simulink model "simulink_guidance_system"  (R2025a)
settings: Solver=VariableStepAuto  StartTime=0.0  StopTime=231  RelTol=1e-3
libraries: slpidlib x1
settings Model: Creator=javia  LastModifiedBy=javia

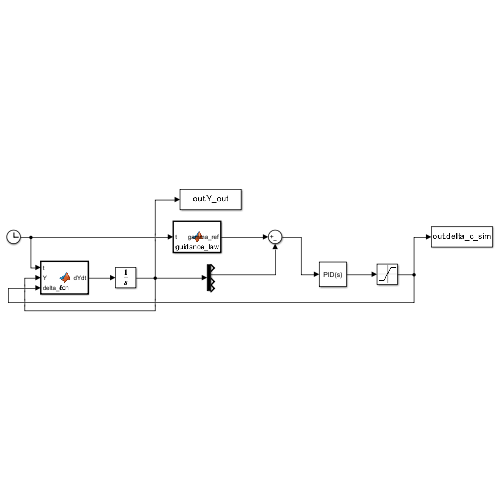
[thumbnail: Simulink's stored preview of the top-level diagram]
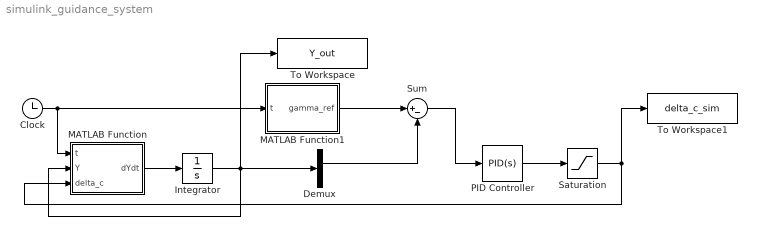
== system simulink_guidance_system ==
  Clock : Clock
  Demux : Demux
  Integrator : Integrator  InitialCondition=[0; pi/2; 0; 0]
  MATLAB Function : MATLAB Function  TreatAsAtomicUnit=on
  MATLAB Function1 : MATLAB Function  TreatAsAtomicUnit=on
  PID Controller : slpidlib/PID Controller  Controller=PID  Form=Parallel  TimeDomain=Continuous-time  UseExternalTs=off  SampleTime=-1  IntegratorMethod=Forward Euler  FilterMethod=Forward Euler  ControllerParametersSource=internal  P=3  I=0.5  UseKiTs=off  D=2  UseExternalDerivativeSource=off  N=100  UseFilter=on  TunerSelectOption=Transfer Function Based (PID Tuner App)  InitialConditionSource=internal  InitialConditionForIntegrator=0  InitialConditionForFilter=0  DifferentiatorICPrevScaledInput=0  ExternalReset=none  TrackingMode=off  Kt=1  LimitOutput=off  SatLimitsSource=internal  UpperSaturationLimit=10 * (pi/180)  LowerSaturationLimit=-10 * (pi/180)  LinearizeAsGain=on  AntiWindupMode=clamping  Kb=1  LimitIntegrator=off  UpperIntegratorSaturationLimit=inf  LowerIntegratorSaturationLimit=-inf  POutMin=[]  POutMax=[]  IOutMin=[]  IOutMax=[]  DOutMin=[]  DOutMax=[]  NOutMin=[]  NOutMax=[]  SumOutMin=[]  SumOutMax=[]  SaturationOutMin=[]  SaturationOutMax=[]  PParamMin=[]  PParamMax=[]  IParamMin=[]  IParamMax=[]  DParamMin=[]  DParamMax=[]  NParamMin=[]  NParamMax=[]  KbParamMin=[]  KbParamMax=[]  KtParamMin=[]  KtParamMax=[]  KbOutMin=[]  KbOutMax=[]  KtOutMin=[]  KtOutMax=[]  IntegratorOutMin=[]  IntegratorOutMax=[]  FilterOutMin=[]  FilterOutMax=[]  SumI1OutMin=[]  SumI1OutMax=[]  SumI2OutMin=[]  SumI2OutMax=[]  SumI3OutMin=[]  SumI3OutMax=[]  SumI4OutMin=[]  SumI4OutMax=[]  SumDOutMin=[]  SumDOutMax=[]  DifferentiatorOutMin=[]  DifferentiatorOutMax=[]  FilterDiffOutCoefMin=[]  FilterDiffOutCoefMax=[]  ReciprocalOutMin=[]  ReciprocalOutMax=[]  SumDenOutMin=[]  SumDenOutMax=[]  SumNumOutMin=[]  SumNumOutMax=[]  DivideOutMin=[]  DivideOutMax=[]  UdiffTsProdOutMin=[]  UdiffTsProdOutMax=[]  NTsProdOutMin=[]  NTsProdOutMax=[]  UintegralTsProdOutMin=[]  UintegralTsProdOutMax=[]  UngainTsProdOutMin=[]  UngainTsProdOutMax=[]  ClampingZeroOutDataTypeStr=Inherit: Inherit via back propagation  ClampingZeroOutMin=[]  ClampingZeroOutMax=[]  FilterDenConstantOutDataTypeStr=Inherit: Inherit via back propagation  FilterDenConstantOutMin=[]  FilterDenConstantOutMax=[]  PCopyOutDataTypeStr=Inherit: Inherit via back propagation  PCopyOutMin=[]  PCopyOutMax=[]  NCopyOutDataTypeStr=Inherit: Inherit via back propagation  NCopyOutMin=[]  NCopyOutMax=[]  IntegratorContinuousStateAttributes=''  IntegratorStateMustResolveToSignalObject=off  IntegratorRTWStateStorageClass=Auto  FilterContinuousStateAttributes=''  FilterStateMustResolveToSignalObject=off  FilterRTWStateStorageClass=Auto  ParallelPVariant=InternalParameters  IdealPVariant=Disabled  IVariant=InternalParameters  DVariant=InternalParameters  IntegratorVariant=Continuous  SatVariant=Disabled  AWVariant=Passthrough  PCopyVariant=Disabled  TRVariant=Disabled  FdbkBlocksVariant=Forward  IdealPFdbkVariant=Disabled  SatFdbkVariant=Disabled  DerivativeFilterVariant=ContFilter  NVariant=InternalParameters  NCopyVariant=Disabled  FilterICVariant=InternalICsFilter  IntegratorICVariant=InternalICs  ExternalResetVariant=Disabled  TRSumVariant=Passthrough  SumFdbkVariant=Disabled  SumVariant=Sum_PID  TsampFilterVariant=InternalTs  TsampNgainVariant=Passthrough  TsampIntegralVariant=Passthrough  ExternalSaturationOutDataTypeStr=Inherit: Same as second input  DerivativeSourceVariant=ErrorSignal  PreIntVariant=InternalPreInt
  Saturation : Saturate  UpperLimit=10 * (pi/180)  LowerLimit=-10 * (pi/180)
  Sum : Sum  Inputs=|+-
  To Workspace : ToWorkspace  VariableName=Y_out  SampleTime=-1
  To Workspace1 : ToWorkspace  VariableName=delta_c_sim  SampleTime=-1
  wires:
  Clock/1 -> MATLAB Function1/1(t), MATLAB Function/1(t)
  MATLAB Function/1(dYdt) -> Integrator/1
  Integrator/1 -> MATLAB Function/2(Y), To Workspace/1, Demux/1
  MATLAB Function1/1(gamma_ref) -> Sum/1
  Demux/2 -> Sum/2
  Sum/1 -> PID Controller/1
  PID Controller/1 -> Saturation/1
  Saturation/1 -> MATLAB Function/3(delta_c), To Workspace1/1

== matlab function simulink_guidance_system/MATLAB Function ==
  data: t input; dYdt output; Y input; delta_c input
function dYdt = fcn(t, Y, delta_c)
    % Obtain current State Vector values
    V = Y(1);
    gamma = Y(2);
    z = Y(3);
    psi = Y(4);
    
    Rt = 6378140;  % Earth mean radius [m]
    
    % Call parameters from your modular files
    [m_t0, tb_1, mass_flow1, T1] = f_stage1();
    [t_GT, ~] = f_gravity_turn();
    [T2, mass_flow2, m0_phase3, tb_2] = f_stage2();
    
    % Calls external function of gravity
    g = f_gravity(z); 
    
    % Calls internal function of aerodynamic drag
    D = f_aerodynamic_drag(Y);
    
    % Calculate the stage and its variables
    if t <= tb_1
        m = m_t0 - mass_flow1 * t;
        T = T1;
    else
        m = m0_phase3 - mass_flow2 * (t - tb_1);
        T = T2;
    end
    
    % Kinematics
    if t <= t_GT
        % PHASE 1: Strictly vertical
        dV_dt = (T - D)/m - g * sin(gamma);  
        dgamma_dt = 0;             
        dz_dt = V * sin(gamma);   
        dpsi_dt = 0;               
    % elseif t > t_GT && t <= t_GT + 1
    %     % THE CONTINUOUS PITCH KICK: Turn maneuver over 1 second
    %     [~, theta_GT] = f_gravity_turn();
    %     dV_dt = (T - D)/m - g * sin(gamma);
    %     dgamma_dt = -theta_GT / 1.0; % Pitch rate [rad/s]
    %     dz_dt = V * sin(gamma);
    %     dpsi_dt = (V * cos(gamma)) / (Rt + z);
    else
        % PHASE 2 & 3: Gravity Turn Kinematics
        % The thrust is decomposed due to the nozzle deflection (delta_c)
        dV_dt = (T*cos(delta_c) - D)/m - g * sin(gamma); 
        % The derivative of gamma is updated according to the nozzle deflection (delta_c)
        dgamma_dt = (T * sin(delta_c) / (m * V)) -(g / V) * cos(gamma) + (V / (Rt + z)) * cos(gamma);  
        dz_dt = V * sin(gamma);   
        dpsi_dt = (V * cos(gamma)) / (Rt + z);               
    end
    
    % Reassemblies derivates in a column vector
    dYdt = [dV_dt; dgamma_dt; dz_dt; dpsi_dt];
end

== matlab function simulink_guidance_system/MATLAB Function1 ==
  data: t input; gamma_ref output
function gamma_ref = guidance_law(t)
    % GUIDANCE COMPUTER: Linear Tangent Steering Law
    
    t_GT = 10;      % Second 10: End of vertical flight clearance
    t_MECO = 231;   % Second 231: Main Engine Cut-Off (End of burn)
    
    if t <= t_GT
        % PHASE 1: Clear the launch pad (strictly vertical)
        gamma_ref = pi/2; 
        
    elseif t > t_MECO
        % PHASE 3: Coasting (keep it horizontal)
        gamma_ref = 0;
        
    else
        % PHASE 2: Optimal Orbital Pitch Over (Linear Tangent Law)
        % We want to transition smoothly from ~90 deg to 0 deg.
        tan_initial = 15; % atan(15) is approx 86.2 degrees
        rate_of_change = tan_initial / (t_MECO - t_GT);
        
        % The magic equation:
        gamma_ref = atan(tan_initial - rate_of_change * (t - t_GT));
    end
end
